simulink model "UAV"  (R2025b)
settings: Solver=ode3  StartTime=0.0  StopTime=inf  FixedStep=Sim.Ts_fisica  RelTol=1e-3
PostLoadFcn:
  | Init
InitFcn:
  | Init
model workspace (MAT data in the model file):
  Mass = 1
undefined symbols (not defined in the file): DiscIntNeverNeededParam, Drone, DWORK0, DWORK1, DWORK10, DWORK11, DWORK12, DWORK13, DWORK14, DWORK15, DWORK16, DWORK17, DWORK18, DWORK19, DWORK2, DWORK20, DWORK21, DWORK22, DWORK23, DWORK24, DWORK3, DWORK4, DWORK5, DWORK6, DWORK7, DWORK8, DWORK9, F, Light, MIL, Sim
libraries: simulink x35, slpidlib x11, vrlib x4, aerolibwind2 x2, sim3dlib x2, uavsim3dlib x2
(part 1 of 8)
settings Model: SimulationMode=accelerator  Creator=1manu  LastModifiedBy=1manu
settings DebuggingCC: InheritedTsInSrcMsg=none

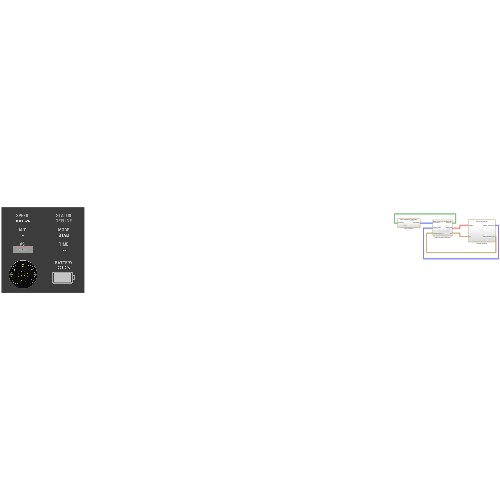
[thumbnail: Simulink's stored preview of the top-level diagram]
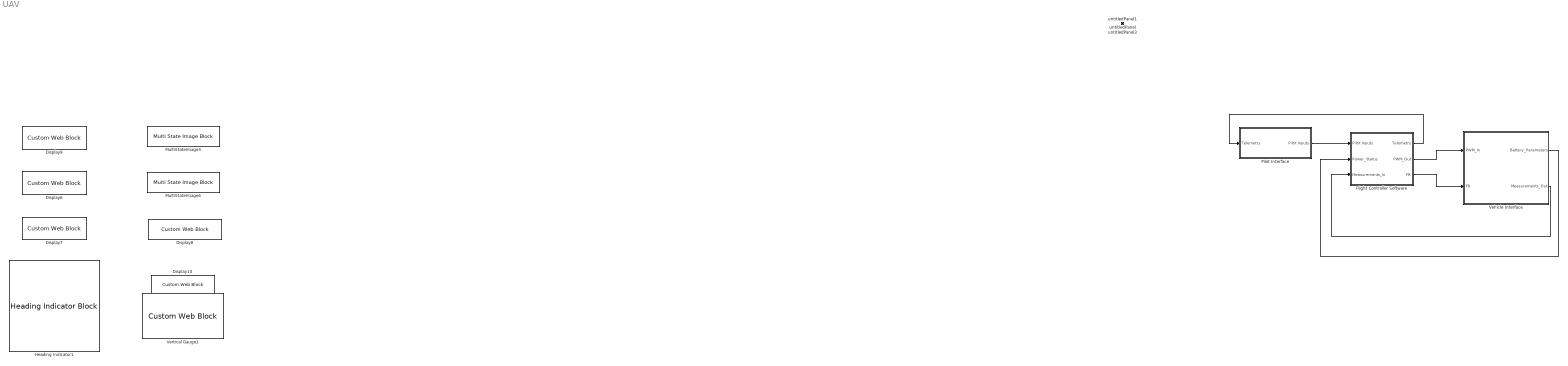
== system UAV ==
  Display10 : CustomWebBlock  LabelPosition=Hide  ShowInitialText=on  Configuration="{\"components\":[{\"name\":\"DisplayComponent\",\"settings\":{\"bold\":true,\"font\":\"Roboto\",\"fontColor\":[255,255,255],\"fontSize\":24,\"format\":\"Custom\",\"formatString\":\"%.1f %%\",\"italic\":false,\"position\":[0,0.005194698952879581,0.9921875,1],\"underline\":false}},{\"name\":\"BackgroundImageComponent\",\"settings\":{\"image\":{\"size\":[160,45],\"src\":\"data:image\\/png;base64,iVBORw0KGgoAAAANSUhEUgAAAKAAAAAtCAIAAACmg\\/d8AAAACXBIWXMAAA7EAAAOxAGVKw4bAAAFRGlUWHRYTUw6Y29tLmFkb2JlLnhtcAAAAAAAPD94cGFja2V0IGJlZ2luPSfvu78nIGlkPSdXNU0wTXBDZWhpSHpyZVN6TlRjemtjOWQnPz4KPHg6eG1wbWV0YSB4bWxuczp4PSdhZG9iZTpuczptZXRhLyc+CjxyZGY6UkRGIHhtbG5zOnJkZj0naHR0cDovL3d3dy53My5vcmcvMTk5OS8wMi8yMi1yZGYtc3ludGF4LW5zIyc+CgogPHJkZjpEZXNjcmlwdGlvbiByZGY6YWJvdXQ9JycKICB4bWxuczpBdHRyaWI9J2h0dHA6Ly9ucy ...(+1822 chars)\",\"srcOrientation\":\"Right\"},\"position\":[0,0,1,1],\"scaleMode\":\"0\"}},{\"name\":\"ForegroundImageComponent\",\"settings\":{\"angle\":0,\"image\":{\"size\":[0,0],\"src\":\"default\"},\"isForeground\":1,\"position\":[0,0,1,1],\"scaleMode\":\"0\"}}],\"derived\":{\"blockParameters\":{\"fixedAspectRatio\":\"on\",\"format\":\"Custom\",\"formatString\":\"%.1f %%\"}},\"settings\":{\"BindingType\":\"signal\",\"aspectRatio\":1.032258064516129,\"backgroundColor\":[0,0,0,\"1\"],\"backgroundOffset\":0.14,\"backgroundOpacity\":1,\"fixedAspectRatio\":\"on\",\"showBackgroundColor\":false,\"value\":0,\"version\":\"R2023b\"},\"type\":\"Display\"}"
  Display6 : CustomWebBlock  LabelPosition=Hide  ShowInitialText=on  Configuration="{\"components\":[{\"name\":\"DisplayComponent\",\"settings\":{\"bold\":true,\"font\":\"Roboto\",\"fontColor\":[255,255,255],\"fontSize\":24,\"format\":\"Custom\",\"formatString\":\"%.1f m\",\"italic\":false,\"position\":[0,0.005194698952879581,0.9921875,1],\"underline\":false}},{\"name\":\"BackgroundImageComponent\",\"settings\":{\"image\":{\"size\":[140,50],\"src\":\"data:image\\/png;base64,iVBORw0KGgoAAAANSUhEUgAAAIwAAAAyCAIAAAABYqRsAAAACXBIWXMAAA7EAAAOxAGVKw4bAAAFU2lUWHRYTUw6Y29tLmFkb2JlLnhtcAAAAAAAPD94cGFja2V0IGJlZ2luPSfvu78nIGlkPSdXNU0wTXBDZWhpSHpyZVN6TlRjemtjOWQnPz4KPHg6eG1wbWV0YSB4bWxuczp4PSdhZG9iZTpuczptZXRhLyc+CjxyZGY6UkRGIHhtbG5zOnJkZj0naHR0cDovL3d3dy53My5vcmcvMTk5OS8wMi8yMi1yZGYtc3ludGF4LW5zIyc+CgogPHJkZjpEZXNjcmlwdGlvbiByZGY6YWJvdXQ9JycKICB4bWxuczpBdHRyaWI9J2h0dHA6Ly9ucy5h ...(+1856 chars)\",\"srcOrientation\":\"Right\"},\"position\":[0,0,1,1],\"scaleMode\":\"0\"}},{\"name\":\"ForegroundImageComponent\",\"settings\":{\"angle\":0,\"image\":{\"size\":[0,0],\"src\":\"default\"},\"isForeground\":1,\"position\":[0,0,1,1],\"scaleMode\":\"0\"}}],\"derived\":{\"blockParameters\":{\"fixedAspectRatio\":\"on\",\"format\":\"Custom\",\"formatString\":\"%.1f m\"}},\"settings\":{\"BindingType\":\"signal\",\"aspectRatio\":1.032258064516129,\"backgroundColor\":[0,0,0,\"1\"],\"backgroundOffset\":0.14,\"backgroundOpacity\":1,\"fixedAspectRatio\":\"on\",\"showBackgroundColor\":false,\"value\":0,\"version\":\"R2023b\"},\"type\":\"Display\"}"
  Display7 : CustomWebBlock  LabelPosition=Hide  ShowInitialText=on  Configuration="{\"components\":[{\"name\":\"DisplayComponent\",\"settings\":{\"bold\":true,\"font\":\"Roboto\",\"fontColor\":[255,255,255],\"fontSize\":24,\"format\":\"Custom\",\"formatString\":\"%.1f m\\/s\",\"italic\":false,\"position\":[0,0.005194698952879581,0.9921875,1],\"underline\":false}},{\"name\":\"BackgroundImageComponent\",\"settings\":{\"image\":{\"size\":[140,50],\"src\":\"data:image\\/png;base64,iVBORw0KGgoAAAANSUhEUgAAAIwAAAAyCAIAAAABYqRsAAAACXBIWXMAAA7EAAAOxAGVKw4bAAAFU2lUWHRYTUw6Y29tLmFkb2JlLnhtcAAAAAAAPD94cGFja2V0IGJlZ2luPSfvu78nIGlkPSdXNU0wTXBDZWhpSHpyZVN6TlRjemtjOWQnPz4KPHg6eG1wbWV0YSB4bWxuczp4PSdhZG9iZTpuczptZXRhLyc+CjxyZGY6UkRGIHhtbG5zOnJkZj0naHR0cDovL3d3dy53My5vcmcvMTk5OS8wMi8yMi1yZGYtc3ludGF4LW5zIyc+CgogPHJkZjpEZXNjcmlwdGlvbiByZGY6YWJvdXQ9JycKICB4bWxuczpBdHRyaWI9J2h0dHA6Ly9ucy5h ...(+1856 chars)\",\"srcOrientation\":\"Right\"},\"position\":[0,0,1,1],\"scaleMode\":\"0\"}},{\"name\":\"ForegroundImageComponent\",\"settings\":{\"angle\":0,\"image\":{\"size\":[0,0],\"src\":\"default\"},\"isForeground\":1,\"position\":[0,0,1,1],\"scaleMode\":\"0\"}}],\"derived\":{\"blockParameters\":{\"fixedAspectRatio\":\"on\",\"format\":\"Custom\",\"formatString\":\"%.1f m\\/s\"}},\"settings\":{\"BindingType\":\"signal\",\"aspectRatio\":1.032258064516129,\"backgroundColor\":[0,0,0,\"1\"],\"backgroundOffset\":0.14,\"backgroundOpacity\":1,\"fixedAspectRatio\":\"on\",\"showBackgroundColor\":false,\"value\":0,\"version\":\"R2023b\"},\"type\":\"Display\"}"
  Display8 : CustomWebBlock  LabelPosition=Hide  ShowInitialText=on  Configuration="{\"components\":[{\"name\":\"DisplayComponent\",\"settings\":{\"bold\":true,\"font\":\"Roboto\",\"fontColor\":[255,255,255],\"fontSize\":24,\"format\":\"Custom\",\"formatString\":\"%.1f\",\"italic\":false,\"position\":[0,0.005194698952879581,0.9921875,1],\"underline\":false}},{\"name\":\"BackgroundImageComponent\",\"settings\":{\"image\":{\"size\":[160,45],\"src\":\"data:image\\/png;base64,iVBORw0KGgoAAAANSUhEUgAAAKAAAAAtCAIAAACmg\\/d8AAAACXBIWXMAAA7EAAAOxAGVKw4bAAAFRGlUWHRYTUw6Y29tLmFkb2JlLnhtcAAAAAAAPD94cGFja2V0IGJlZ2luPSfvu78nIGlkPSdXNU0wTXBDZWhpSHpyZVN6TlRjemtjOWQnPz4KPHg6eG1wbWV0YSB4bWxuczp4PSdhZG9iZTpuczptZXRhLyc+CjxyZGY6UkRGIHhtbG5zOnJkZj0naHR0cDovL3d3dy53My5vcmcvMTk5OS8wMi8yMi1yZGYtc3ludGF4LW5zIyc+CgogPHJkZjpEZXNjcmlwdGlvbiByZGY6YWJvdXQ9JycKICB4bWxuczpBdHRyaWI9J2h0dHA6Ly9ucy ...(+1822 chars)\",\"srcOrientation\":\"Right\"},\"position\":[0,0,1,1],\"scaleMode\":\"0\"}},{\"name\":\"ForegroundImageComponent\",\"settings\":{\"angle\":0,\"image\":{\"size\":[0,0],\"src\":\"default\"},\"isForeground\":1,\"position\":[0,0,1,1],\"scaleMode\":\"0\"}}],\"derived\":{\"blockParameters\":{\"fixedAspectRatio\":\"on\",\"format\":\"Custom\",\"formatString\":\"%.1f\"}},\"settings\":{\"BindingType\":\"signal\",\"aspectRatio\":1.032258064516129,\"backgroundColor\":[0,0,0,\"1\"],\"backgroundOffset\":0.14,\"backgroundOpacity\":1,\"fixedAspectRatio\":\"on\",\"showBackgroundColor\":false,\"value\":0,\"version\":\"R2023b\"},\"type\":\"Display\"}"
  Display9 : CustomWebBlock  LabelPosition=Hide  ShowInitialText=on  Configuration="{\"components\":[{\"name\":\"DisplayComponent\",\"settings\":{\"bold\":true,\"font\":\"Roboto\",\"fontColor\":[255,255,255],\"fontSize\":24,\"format\":\"Custom\",\"formatString\":\"%.1f km\\/h\",\"italic\":false,\"position\":[0,0.005194698952879581,0.9921875,1],\"underline\":false}},{\"name\":\"BackgroundImageComponent\",\"settings\":{\"image\":{\"size\":[140,50],\"src\":\"data:image\\/png;base64,iVBORw0KGgoAAAANSUhEUgAAAIwAAAAyCAIAAAABYqRsAAAACXBIWXMAAA7EAAAOxAGVKw4bAAAFU2lUWHRYTUw6Y29tLmFkb2JlLnhtcAAAAAAAPD94cGFja2V0IGJlZ2luPSfvu78nIGlkPSdXNU0wTXBDZWhpSHpyZVN6TlRjemtjOWQnPz4KPHg6eG1wbWV0YSB4bWxuczp4PSdhZG9iZTpuczptZXRhLyc+CjxyZGY6UkRGIHhtbG5zOnJkZj0naHR0cDovL3d3dy53My5vcmcvMTk5OS8wMi8yMi1yZGYtc3ludGF4LW5zIyc+CgogPHJkZjpEZXNjcmlwdGlvbiByZGY6YWJvdXQ9JycKICB4bWxuczpBdHRyaWI9J2h0dHA6Ly9ucy5h ...(+1856 chars)\",\"srcOrientation\":\"Right\"},\"position\":[0,0,1,1],\"scaleMode\":\"0\"}},{\"name\":\"ForegroundImageComponent\",\"settings\":{\"angle\":0,\"image\":{\"size\":[0,0],\"src\":\"default\"},\"isForeground\":1,\"position\":[0,0,1,1],\"scaleMode\":\"0\"}}],\"derived\":{\"blockParameters\":{\"fixedAspectRatio\":\"on\",\"format\":\"Custom\",\"formatString\":\"%.1f km\\/h\"}},\"settings\":{\"BindingType\":\"signal\",\"aspectRatio\":1.032258064516129,\"backgroundColor\":[0,0,0,\"1\"],\"backgroundOffset\":0.14,\"backgroundOpacity\":1,\"fixedAspectRatio\":\"on\",\"showBackgroundColor\":false,\"value\":0,\"version\":\"R2023b\"},\"type\":\"Display\"}"
  Flight Controller Software : Subsystem  Variant=on
  Heading Indicator1 : HeadingIndicatorBlock  LabelPosition=Hide
  MultiStateImage3 : MultiStateImageBlock  LabelPosition=Hide
  MultiStateImage4 : MultiStateImageBlock  LabelPosition=Hide
  Pilot Interface : Subsystem  Variant=on  EmptyChoice=on
  Vehicle Interface : Subsystem  Variant=on  EmptyChoice=on
  Vertical Gauge1 : CustomWebBlock  LabelPosition=Hide  ShowInitialText=on  Configuration="{\"components\":[{\"name\":\"LinearScaleComponent\",\"settings\":{\"bounds\":{\"max\":100,\"min\":0,\"tickInterval\":\"auto\"},\"internalTickHeightScaleFactor\":1.6,\"labelColor\":[128,128,128],\"labelFont\":{\"font\":\"Arial\",\"fontSize\":12},\"labelOffset\":0.05,\"labelTransparency\":1,\"needleImage\":{\"size\":[0,0],\"src\":\"\"},\"needleOffset\":[0,0],\"needleSize\":{\"height\":0,\"width\":0},\"position\":[0.19205729166666666,0.08571428571428574,0.7442857142857143,0.6202799479166666],\"referencePoint\":\"auto\",\"scaleColors\":[],\"scaleColorsSize\":0.2,\"scaleDirection\":\"LR\",\"showLabels\":false,\"showMinorTicks\":0,\"showSpanLine\":false,\"showTicks\":false,\"tickColor\":[0,0,0],\"tickTransparency\":0.7,\"valueBarColor\":[230,230,230],\"valueBarOffset\":-0.09,\"valueBarSize\":0.96,\"valueBarTransparency\":1}},{\"name\":\"BackgroundImageComponent\",\"settings\":{\"image\":{\"size\":[232,418],\"src\":\"data:image\\/png;base64,iVBORw0KGgoAAAANSUhEUgAAAOgAAAGiCAYAAADtHYrGAAAAAXNSR0IArs4c6QAAAARnQU1BAACxjwv8YQUAAAAJcEhZcwAACxAAAAsQAa0jvXUAAAC0ZVhJZklJKgAIAAAABgASAQMAAQAAAAEAAAAaAQUAAQAAAFYAAAAbAQUAAQAAAF4AAAAoAQMAAQAAAAIAAAATAgMAAQAAAAEAAABphwQAAQAAAGYAAAAAAAAASAAAAAEAAABIAAAAAQAAAAYAAJAHAAQAAAAwMjEwAZEHAAQAAAABAgMAAKAHAAQAAAAwMTAwAaADAAEAAAD\\/\\/wAAAqAEAAEAAAAAAgAAA6AEAAEAAAAAAgAAAAAAAJFf8doAAAGHaVRYdFhNTDpjb20uYWRvYmUu ...(+3414 chars)\",\"srcOrientation\":\"Up\"},\"position\":[0,0,1,1],\"scaleMode\":\"0\"}},{\"name\":\"ForegroundImageComponent\",\"settings\":{\"image\":{\"size\":[0,0],\"src\":\"default\",\"srcOrientation\":[]},\"isForeground\":1,\"position\":[0,0,1,1],\"scaleMode\":\"0\"}}],\"derived\":{\"blockParameters\":{\"ForegroundColor\":[0,0,0],\"Limits\":{\"Max\":100,\"Min\":0,\"Ticks\":\"auto\"},\"ScaleColors\":[],\"ScaleDirection\":\"Clockwise\",\"ScaleMax\":100,\"ScaleMin\":0,\"TickInterval\":\"auto\",\"fixedAspectRatio\":\"on\"}},\"settings\":{\"BindingType\":\"signal\",\"backgroundColor\":[0,0,0,\"1\"],\"backgroundOffset\":0,\"backgroundOpacity\":1,\"fixedAspectRatio\":\"on\",\"orientation\":\"horizontal\",\"showBackgroundColor\":false,\"value\":0,\"version\":\"R2023a\"},\"type\":\"LinearGauge\"}"  CustomBackgroundColor="{\"color\":[0.8,0.8,0.8],\"show\":false}"
  untitledPanel : Subsystem  Tag=HiddenForWebPanel  IsWebBlockPanel=on
  untitledPanel1 : Subsystem  Tag=HiddenForWebPanel  IsWebBlockPanel=on
  untitledPanel3 : Subsystem  Tag=HiddenForWebPanel  IsWebBlockPanel=on
  wires:
  Pilot Interface/1(Pilot Inputs) -> Flight Controller Software/1(Pilot Inputs)
  Vehicle Interface/1(Battery_Parameters) -> Flight Controller Software/2(Power_Status)
  Vehicle Interface/2(Measurements_Out) -> Flight Controller Software/3(Measurements_In)
  Flight Controller Software/1("Telemetry ") -> Pilot Interface/1("Telemetry ")
  Flight Controller Software/2(PWM_Out) -> Vehicle Interface/1(PWM_In)
  Flight Controller Software/3(FR) -> Vehicle Interface/2(FR)

== system UAV/Flight Controller Software ==
  Pilot Inputs : Inport
  Power_Status : Inport  Port=2
  Measurements_In : Inport  Port=3
  Flight Controller Software MIL : Subsystem  TreatAsAtomicUnit=on  VariantControl=SIL_MODE == 0
  Flight Controller Software SIL : Subsystem  VariantControl=SIL_MODE == 1
      mask help: Simulink:masks:GenSFuncDesc_MD
      mask Help: eval('feval(''rtwprivate'',''rtwhelpview'',''rtw_sfcn_block'')');
  "Telemetry " : Outport
  PWM_Out : Outport  Port=2
  FR : Outport  Port=3

== system UAV/Pilot Interface ==
  "Telemetry " : Inport
  "Real_Receiver_Driver " : Subsystem  VariantControl=HIL_MODE==1
  "SIM_Flightstick_HotasX56 " : Subsystem  VariantControl=HIL_MODE==0
  Pilot Inputs : Outport

== system UAV/Vehicle Interface ==
  PWM_In : Inport
  FR : Inport  Port=2
  Real_Hardware_Drivers : Subsystem  VariantControl=HIL_MODE == 1
  Sim_Plant_Model : Subsystem  VariantControl=HIL_MODE == 0
  Battery_Parameters : Outport
  Measurements_Out : Outport  Port=2
